simulink model "lab4_test"  (R2016b)
settings: Solver=VariableStepAuto  StartTime=0.0  StopTime=totaltime  RelTol=1e-3
undefined symbols (not defined in the file or in its folder): h, st
libraries: xbsIndex_r4 x1157
(part 2 of 3)

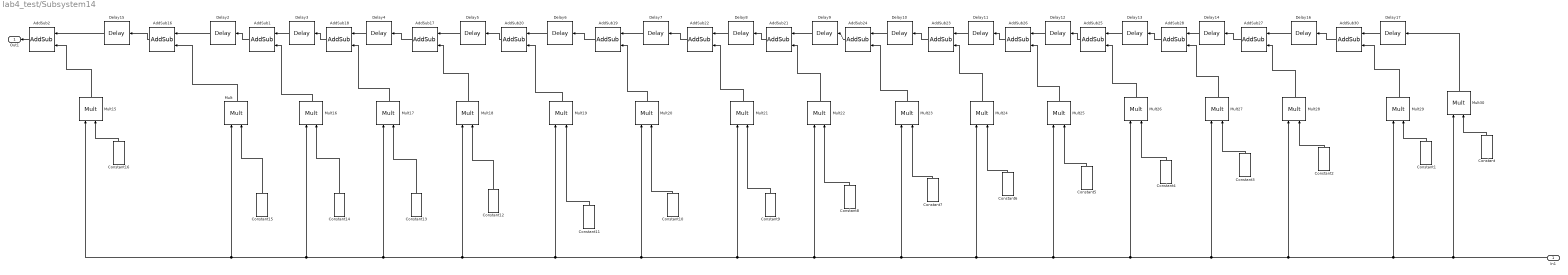
== system lab4_test/Subsystem14 ==
  In1 : Inport
  AddSub{1..2,16..28,30} (16 alike) : xbsIndex_r4/AddSub  mode=Addition  use_carryin=off  use_carryout=off  en=off  latency=0  precision=User Defined  arith_type="Signed  (2's comp)"  n_bits=W  bin_pt=B  quantization=Truncate  overflow=Wrap  use_behavioral_HDL=off  hw_selection=Fabric  pipelined=off  dbl_ovrd=off  block_type=addsub
  Constant : xbsIndex_r4/Constant  const=h(1,4)  gui_display_data_type=Fixed-point  arith_type=Signed (2's comp)  n_bits=W  bin_pt=B  preci_type=Single  exp_width=8  frac_width=24  explicit_period=off  period=1  equ=P=C  opselect=C  inp2=PCIN>>17  opr=+  inp1=P  carry=CIN  dbl_ovrd=off  block_type=constant
  Constant1 : xbsIndex_r4/Constant  const=h(2,4)  gui_display_data_type=Fixed-point  arith_type=Signed (2's comp)  n_bits=W  bin_pt=B  preci_type=Single  exp_width=8  frac_width=24  explicit_period=off  period=1  equ=P=C  opselect=C  inp2=PCIN>>17  opr=+  inp1=P  carry=CIN  dbl_ovrd=off  block_type=constant
  Constant10 : xbsIndex_r4/Constant  const=h(11,4)  gui_display_data_type=Fixed-point  arith_type=Signed (2's comp)  n_bits=W  bin_pt=B  preci_type=Single  exp_width=8  frac_width=24  explicit_period=off  period=1  equ=P=C  opselect=C  inp2=PCIN>>17  opr=+  inp1=P  carry=CIN  dbl_ovrd=off  block_type=constant
  Constant11 : xbsIndex_r4/Constant  const=h(12,4)  gui_display_data_type=Fixed-point  arith_type=Signed (2's comp)  n_bits=W  bin_pt=B  preci_type=Single  exp_width=8  frac_width=24  explicit_period=off  period=1  equ=P=C  opselect=C  inp2=PCIN>>17  opr=+  inp1=P  carry=CIN  dbl_ovrd=off  block_type=constant
  Constant12 : xbsIndex_r4/Constant  const=h(13,4)  gui_display_data_type=Fixed-point  arith_type=Signed (2's comp)  n_bits=W  bin_pt=B  preci_type=Single  exp_width=8  frac_width=24  explicit_period=off  period=1  equ=P=C  opselect=C  inp2=PCIN>>17  opr=+  inp1=P  carry=CIN  dbl_ovrd=off  block_type=constant
  Constant13 : xbsIndex_r4/Constant  const=h(14,4)  gui_display_data_type=Fixed-point  arith_type=Signed (2's comp)  n_bits=W  bin_pt=B  preci_type=Single  exp_width=8  frac_width=24  explicit_period=off  period=1  equ=P=C  opselect=C  inp2=PCIN>>17  opr=+  inp1=P  carry=CIN  dbl_ovrd=off  block_type=constant
  Constant14 : xbsIndex_r4/Constant  const=h(15,4)  gui_display_data_type=Fixed-point  arith_type=Signed (2's comp)  n_bits=W  bin_pt=B  preci_type=Single  exp_width=8  frac_width=24  explicit_period=off  period=1  equ=P=C  opselect=C  inp2=PCIN>>17  opr=+  inp1=P  carry=CIN  dbl_ovrd=off  block_type=constant
  Constant15 : xbsIndex_r4/Constant  const=h(16,4)  gui_display_data_type=Fixed-point  arith_type=Signed (2's comp)  n_bits=W  bin_pt=B  preci_type=Single  exp_width=8  frac_width=24  explicit_period=off  period=1  equ=P=C  opselect=C  inp2=PCIN>>17  opr=+  inp1=P  carry=CIN  dbl_ovrd=off  block_type=constant
  Constant16 : xbsIndex_r4/Constant  const=h(17,4)  gui_display_data_type=Fixed-point  arith_type=Signed (2's comp)  n_bits=W  bin_pt=B  preci_type=Single  exp_width=8  frac_width=24  explicit_period=off  period=1  equ=P=C  opselect=C  inp2=PCIN>>17  opr=+  inp1=P  carry=CIN  dbl_ovrd=off  block_type=constant
  Constant2 : xbsIndex_r4/Constant  const=h(3,4)  gui_display_data_type=Fixed-point  arith_type=Signed (2's comp)  n_bits=W  bin_pt=B  preci_type=Single  exp_width=8  frac_width=24  explicit_period=off  period=1  equ=P=C  opselect=C  inp2=PCIN>>17  opr=+  inp1=P  carry=CIN  dbl_ovrd=off  block_type=constant
  Constant3 : xbsIndex_r4/Constant  const=h(4,4)  gui_display_data_type=Fixed-point  arith_type=Signed (2's comp)  n_bits=W  bin_pt=B  preci_type=Single  exp_width=8  frac_width=24  explicit_period=off  period=1  equ=P=C  opselect=C  inp2=PCIN>>17  opr=+  inp1=P  carry=CIN  dbl_ovrd=off  block_type=constant
  Constant4 : xbsIndex_r4/Constant  const=h(5,4)  gui_display_data_type=Fixed-point  arith_type=Signed (2's comp)  n_bits=W  bin_pt=B  preci_type=Single  exp_width=8  frac_width=24  explicit_period=off  period=1  equ=P=C  opselect=C  inp2=PCIN>>17  opr=+  inp1=P  carry=CIN  dbl_ovrd=off  block_type=constant
  Constant5 : xbsIndex_r4/Constant  const=h(6,4)  gui_display_data_type=Fixed-point  arith_type=Signed (2's comp)  n_bits=W  bin_pt=B  preci_type=Single  exp_width=8  frac_width=24  explicit_period=off  period=1  equ=P=C  opselect=C  inp2=PCIN>>17  opr=+  inp1=P  carry=CIN  dbl_ovrd=off  block_type=constant
  Constant6 : xbsIndex_r4/Constant  const=h(7,4)  gui_display_data_type=Fixed-point  arith_type=Signed (2's comp)  n_bits=W  bin_pt=B  preci_type=Single  exp_width=8  frac_width=24  explicit_period=off  period=1  equ=P=C  opselect=C  inp2=PCIN>>17  opr=+  inp1=P  carry=CIN  dbl_ovrd=off  block_type=constant
  Constant7 : xbsIndex_r4/Constant  const=h(8,4)  gui_display_data_type=Fixed-point  arith_type=Signed (2's comp)  n_bits=W  bin_pt=B  preci_type=Single  exp_width=8  frac_width=24  explicit_period=off  period=1  equ=P=C  opselect=C  inp2=PCIN>>17  opr=+  inp1=P  carry=CIN  dbl_ovrd=off  block_type=constant
  Constant8 : xbsIndex_r4/Constant  const=h(9,4)  gui_display_data_type=Fixed-point  arith_type=Signed (2's comp)  n_bits=W  bin_pt=B  preci_type=Single  exp_width=8  frac_width=24  explicit_period=off  period=1  equ=P=C  opselect=C  inp2=PCIN>>17  opr=+  inp1=P  carry=CIN  dbl_ovrd=off  block_type=constant
  Constant9 : xbsIndex_r4/Constant  const=h(10,4)  gui_display_data_type=Fixed-point  arith_type=Signed (2's comp)  n_bits=W  bin_pt=B  preci_type=Single  exp_width=8  frac_width=24  explicit_period=off  period=1  equ=P=C  opselect=C  inp2=PCIN>>17  opr=+  inp1=P  carry=CIN  dbl_ovrd=off  block_type=constant
  Delay{2..17} (16 alike) : xbsIndex_r4/Delay  rst=off  infoeditControl=Selection of Reset will increase slice count due to use of real FFs and instead of SRLs  en=off  latency=1  reg_retiming=off  dbl_ovrd=off  block_type=delay
  Mult{,15..30} (17 alike) : xbsIndex_r4/Mult  precision=User Defined  arith_type="Signed  (2's comp)"  n_bits=W  bin_pt=B  quantization="Round  (unbiased: +/- Inf)"  overflow=Flag as error  en=off  latency=0  use_behavioral_HDL=off  opt=Speed  use_embedded=on  optimum_pipeline=off  pipeline=on  dbl_ovrd=off  use_rpm=on  placement_style=Triangular  block_type=mult
  Out1 : Outport
  wires:
  AddSub2/1 -> Out1/1
  Constant14/1 -> Mult16/2
  Mult/1 -> AddSub16/2
  Mult16/1 -> AddSub1/2
  AddSub16/1 -> Delay15/1
  Constant15/1 -> Mult/2
  AddSub1/1 -> Delay2/1
  Constant13/1 -> Mult17/2
  Mult17/1 -> AddSub18/2
  Constant12/1 -> Mult18/2
  AddSub17/1 -> Delay4/1
  AddSub18/1 -> Delay3/1
  Constant11/1 -> Mult19/2
  Mult19/1 -> AddSub20/2
  Constant10/1 -> Mult20/2
  Mult20/1 -> AddSub19/2
  AddSub19/1 -> Delay6/1
  AddSub20/1 -> Delay5/1
  Constant9/1 -> Mult21/2
  Mult21/1 -> AddSub22/2
  Constant8/1 -> Mult22/2
  AddSub21/1 -> Delay8/1
  AddSub22/1 -> Delay7/1
  Constant7/1 -> Mult23/2
  Mult23/1 -> AddSub24/2
  Constant6/1 -> Mult24/2
  AddSub23/1 -> Delay10/1
  Constant5/1 -> Mult25/2
  Mult25/1 -> AddSub26/2
  Constant4/1 -> Mult26/2
  Mult26/1 -> AddSub25/2
  AddSub25/1 -> Delay12/1
  AddSub26/1 -> Delay11/1
  Constant3/1 -> Mult27/2
  Mult27/1 -> AddSub28/2
  Constant2/1 -> Mult28/2
  AddSub27/1 -> Delay14/1
  AddSub28/1 -> Delay13/1
  Constant1/1 -> Mult29/2
  Mult29/1 -> AddSub30/2
  Constant/1 -> Mult30/2
  Mult30/1 -> Delay17/1
  AddSub30/1 -> Delay16/1
  AddSub24/1 -> Delay9/1
  Delay2/1 -> AddSub16/1
  Delay3/1 -> AddSub1/1
  Delay4/1 -> AddSub18/1
  Delay6/1 -> AddSub20/1
  Delay7/1 -> AddSub19/1
  Delay8/1 -> AddSub22/1
  Delay10/1 -> AddSub24/1
  Delay12/1 -> AddSub26/1
  Delay13/1 -> AddSub25/1
  Delay14/1 -> AddSub28/1
  Delay17/1 -> AddSub30/1
  Constant16/1 -> Mult15/2
  Mult15/1 -> AddSub2/2
  Delay15/1 -> AddSub2/1
  Delay5/1 -> AddSub17/1
  Mult18/1 -> AddSub17/2
  Delay9/1 -> AddSub21/1
  Mult22/1 -> AddSub21/2
  Delay11/1 -> AddSub23/1
  Mult24/1 -> AddSub23/2
  Delay16/1 -> AddSub27/1
  Mult28/1 -> AddSub27/2
  In1/1 -> Mult30/1, Mult29/1, Mult28/1, Mult27/1, Mult26/1, Mult25/1, Mult24/1, Mult22/1, Mult21/1, Mult19/1, Mult17/1, Mult15/1, Mult/1, Mult16/1, Mult18/1, Mult20/1, Mult23/1

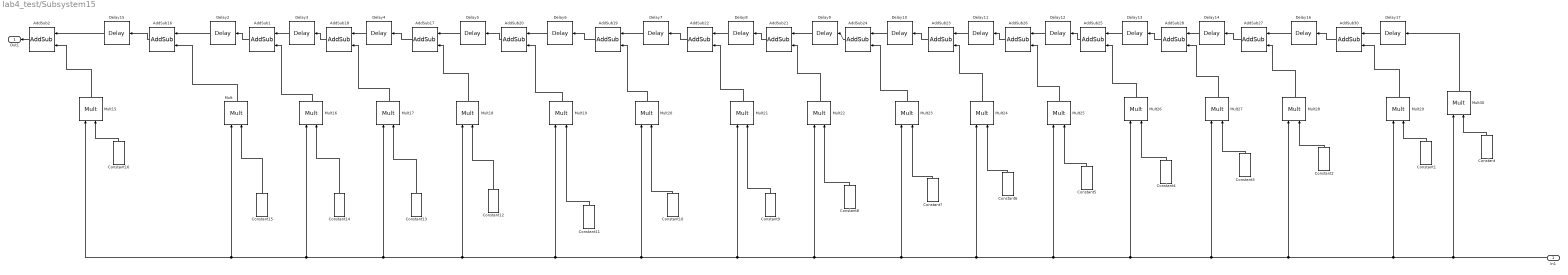
== system lab4_test/Subsystem15 ==
  In1 : Inport
  AddSub{1..2,16..28,30} (16 alike) : xbsIndex_r4/AddSub  mode=Addition  use_carryin=off  use_carryout=off  en=off  latency=0  precision=User Defined  arith_type="Signed  (2's comp)"  n_bits=W  bin_pt=B  quantization=Truncate  overflow=Wrap  use_behavioral_HDL=off  hw_selection=Fabric  pipelined=off  dbl_ovrd=off  block_type=addsub
  Constant : xbsIndex_r4/Constant  const=h(1,3)  gui_display_data_type=Fixed-point  arith_type=Signed (2's comp)  n_bits=W  bin_pt=B  preci_type=Single  exp_width=8  frac_width=24  explicit_period=off  period=1  equ=P=C  opselect=C  inp2=PCIN>>17  opr=+  inp1=P  carry=CIN  dbl_ovrd=off  block_type=constant
  Constant1 : xbsIndex_r4/Constant  const=h(2,3)  gui_display_data_type=Fixed-point  arith_type=Signed (2's comp)  n_bits=W  bin_pt=B  preci_type=Single  exp_width=8  frac_width=24  explicit_period=off  period=1  equ=P=C  opselect=C  inp2=PCIN>>17  opr=+  inp1=P  carry=CIN  dbl_ovrd=off  block_type=constant
  Constant10 : xbsIndex_r4/Constant  const=h(11,3)  gui_display_data_type=Fixed-point  arith_type=Signed (2's comp)  n_bits=W  bin_pt=B  preci_type=Single  exp_width=8  frac_width=24  explicit_period=off  period=1  equ=P=C  opselect=C  inp2=PCIN>>17  opr=+  inp1=P  carry=CIN  dbl_ovrd=off  block_type=constant
  Constant11 : xbsIndex_r4/Constant  const=h(12,3)  gui_display_data_type=Fixed-point  arith_type=Signed (2's comp)  n_bits=W  bin_pt=B  preci_type=Single  exp_width=8  frac_width=24  explicit_period=off  period=1  equ=P=C  opselect=C  inp2=PCIN>>17  opr=+  inp1=P  carry=CIN  dbl_ovrd=off  block_type=constant
  Constant12 : xbsIndex_r4/Constant  const=h(13,3)  gui_display_data_type=Fixed-point  arith_type=Signed (2's comp)  n_bits=W  bin_pt=B  preci_type=Single  exp_width=8  frac_width=24  explicit_period=off  period=1  equ=P=C  opselect=C  inp2=PCIN>>17  opr=+  inp1=P  carry=CIN  dbl_ovrd=off  block_type=constant
  Constant13 : xbsIndex_r4/Constant  const=h(14,3)  gui_display_data_type=Fixed-point  arith_type=Signed (2's comp)  n_bits=W  bin_pt=B  preci_type=Single  exp_width=8  frac_width=24  explicit_period=off  period=1  equ=P=C  opselect=C  inp2=PCIN>>17  opr=+  inp1=P  carry=CIN  dbl_ovrd=off  block_type=constant
  Constant14 : xbsIndex_r4/Constant  const=h(15,3)  gui_display_data_type=Fixed-point  arith_type=Signed (2's comp)  n_bits=W  bin_pt=B  preci_type=Single  exp_width=8  frac_width=24  explicit_period=off  period=1  equ=P=C  opselect=C  inp2=PCIN>>17  opr=+  inp1=P  carry=CIN  dbl_ovrd=off  block_type=constant
  Constant15 : xbsIndex_r4/Constant  const=h(16,3)  gui_display_data_type=Fixed-point  arith_type=Signed (2's comp)  n_bits=W  bin_pt=B  preci_type=Single  exp_width=8  frac_width=24  explicit_period=off  period=1  equ=P=C  opselect=C  inp2=PCIN>>17  opr=+  inp1=P  carry=CIN  dbl_ovrd=off  block_type=constant
  Constant16 : xbsIndex_r4/Constant  const=h(17,3)  gui_display_data_type=Fixed-point  arith_type=Signed (2's comp)  n_bits=W  bin_pt=B  preci_type=Single  exp_width=8  frac_width=24  explicit_period=off  period=1  equ=P=C  opselect=C  inp2=PCIN>>17  opr=+  inp1=P  carry=CIN  dbl_ovrd=off  block_type=constant
  Constant2 : xbsIndex_r4/Constant  const=h(3,3)  gui_display_data_type=Fixed-point  arith_type=Signed (2's comp)  n_bits=W  bin_pt=B  preci_type=Single  exp_width=8  frac_width=24  explicit_period=off  period=1  equ=P=C  opselect=C  inp2=PCIN>>17  opr=+  inp1=P  carry=CIN  dbl_ovrd=off  block_type=constant
  Constant3 : xbsIndex_r4/Constant  const=h(4,3)  gui_display_data_type=Fixed-point  arith_type=Signed (2's comp)  n_bits=W  bin_pt=B  preci_type=Single  exp_width=8  frac_width=24  explicit_period=off  period=1  equ=P=C  opselect=C  inp2=PCIN>>17  opr=+  inp1=P  carry=CIN  dbl_ovrd=off  block_type=constant
  Constant4 : xbsIndex_r4/Constant  const=h(5,3)  gui_display_data_type=Fixed-point  arith_type=Signed (2's comp)  n_bits=W  bin_pt=B  preci_type=Single  exp_width=8  frac_width=24  explicit_period=off  period=1  equ=P=C  opselect=C  inp2=PCIN>>17  opr=+  inp1=P  carry=CIN  dbl_ovrd=off  block_type=constant
  Constant5 : xbsIndex_r4/Constant  const=h(6,3)  gui_display_data_type=Fixed-point  arith_type=Signed (2's comp)  n_bits=W  bin_pt=B  preci_type=Single  exp_width=8  frac_width=24  explicit_period=off  period=1  equ=P=C  opselect=C  inp2=PCIN>>17  opr=+  inp1=P  carry=CIN  dbl_ovrd=off  block_type=constant
  Constant6 : xbsIndex_r4/Constant  const=h(7,3)  gui_display_data_type=Fixed-point  arith_type=Signed (2's comp)  n_bits=W  bin_pt=B  preci_type=Single  exp_width=8  frac_width=24  explicit_period=off  period=1  equ=P=C  opselect=C  inp2=PCIN>>17  opr=+  inp1=P  carry=CIN  dbl_ovrd=off  block_type=constant
  Constant7 : xbsIndex_r4/Constant  const=h(8,3)  gui_display_data_type=Fixed-point  arith_type=Signed (2's comp)  n_bits=W  bin_pt=B  preci_type=Single  exp_width=8  frac_width=24  explicit_period=off  period=1  equ=P=C  opselect=C  inp2=PCIN>>17  opr=+  inp1=P  carry=CIN  dbl_ovrd=off  block_type=constant
  Constant8 : xbsIndex_r4/Constant  const=h(9,3)  gui_display_data_type=Fixed-point  arith_type=Signed (2's comp)  n_bits=W  bin_pt=B  preci_type=Single  exp_width=8  frac_width=24  explicit_period=off  period=1  equ=P=C  opselect=C  inp2=PCIN>>17  opr=+  inp1=P  carry=CIN  dbl_ovrd=off  block_type=constant
  Constant9 : xbsIndex_r4/Constant  const=h(10,3)  gui_display_data_type=Fixed-point  arith_type=Signed (2's comp)  n_bits=W  bin_pt=B  preci_type=Single  exp_width=8  frac_width=24  explicit_period=off  period=1  equ=P=C  opselect=C  inp2=PCIN>>17  opr=+  inp1=P  carry=CIN  dbl_ovrd=off  block_type=constant
  Delay{2..17} (16 alike) : xbsIndex_r4/Delay  rst=off  infoeditControl=Selection of Reset will increase slice count due to use of real FFs and instead of SRLs  en=off  latency=1  reg_retiming=off  dbl_ovrd=off  block_type=delay
  Mult{,15..30} (17 alike) : xbsIndex_r4/Mult  precision=User Defined  arith_type="Signed  (2's comp)"  n_bits=W  bin_pt=B  quantization="Round  (unbiased: +/- Inf)"  overflow=Flag as error  en=off  latency=0  use_behavioral_HDL=off  opt=Speed  use_embedded=on  optimum_pipeline=off  pipeline=on  dbl_ovrd=off  use_rpm=on  placement_style=Triangular  block_type=mult
  Out1 : Outport
  wires:
  AddSub2/1 -> Out1/1
  Constant14/1 -> Mult16/2
  Mult/1 -> AddSub16/2
  Mult16/1 -> AddSub1/2
  AddSub16/1 -> Delay15/1
  Constant15/1 -> Mult/2
  AddSub1/1 -> Delay2/1
  Constant13/1 -> Mult17/2
  Mult17/1 -> AddSub18/2
  Constant12/1 -> Mult18/2
  AddSub17/1 -> Delay4/1
  AddSub18/1 -> Delay3/1
  Constant11/1 -> Mult19/2
  Mult19/1 -> AddSub20/2
  Constant10/1 -> Mult20/2
  Mult20/1 -> AddSub19/2
  AddSub19/1 -> Delay6/1
  AddSub20/1 -> Delay5/1
  Constant9/1 -> Mult21/2
  Mult21/1 -> AddSub22/2
  Constant8/1 -> Mult22/2
  AddSub21/1 -> Delay8/1
  AddSub22/1 -> Delay7/1
  Constant7/1 -> Mult23/2
  Mult23/1 -> AddSub24/2
  Constant6/1 -> Mult24/2
  AddSub23/1 -> Delay10/1
  Constant5/1 -> Mult25/2
  Mult25/1 -> AddSub26/2
  Constant4/1 -> Mult26/2
  Mult26/1 -> AddSub25/2
  AddSub25/1 -> Delay12/1
  AddSub26/1 -> Delay11/1
  Constant3/1 -> Mult27/2
  Mult27/1 -> AddSub28/2
  Constant2/1 -> Mult28/2
  AddSub27/1 -> Delay14/1
  AddSub28/1 -> Delay13/1
  Constant1/1 -> Mult29/2
  Mult29/1 -> AddSub30/2
  Constant/1 -> Mult30/2
  Mult30/1 -> Delay17/1
  AddSub30/1 -> Delay16/1
  AddSub24/1 -> Delay9/1
  Delay2/1 -> AddSub16/1
  Delay3/1 -> AddSub1/1
  Delay4/1 -> AddSub18/1
  Delay6/1 -> AddSub20/1
  Delay7/1 -> AddSub19/1
  Delay8/1 -> AddSub22/1
  Delay10/1 -> AddSub24/1
  Delay12/1 -> AddSub26/1
  Delay13/1 -> AddSub25/1
  Delay14/1 -> AddSub28/1
  Delay17/1 -> AddSub30/1
  Constant16/1 -> Mult15/2
  Mult15/1 -> AddSub2/2
  Delay15/1 -> AddSub2/1
  Delay5/1 -> AddSub17/1
  Mult18/1 -> AddSub17/2
  Delay9/1 -> AddSub21/1
  Mult22/1 -> AddSub21/2
  Delay11/1 -> AddSub23/1
  Mult24/1 -> AddSub23/2
  Delay16/1 -> AddSub27/1
  Mult28/1 -> AddSub27/2
  In1/1 -> Mult30/1, Mult29/1, Mult28/1, Mult27/1, Mult26/1, Mult25/1, Mult24/1, Mult22/1, Mult21/1, Mult19/1, Mult17/1, Mult15/1, Mult/1, Mult16/1, Mult18/1, Mult20/1, Mult23/1

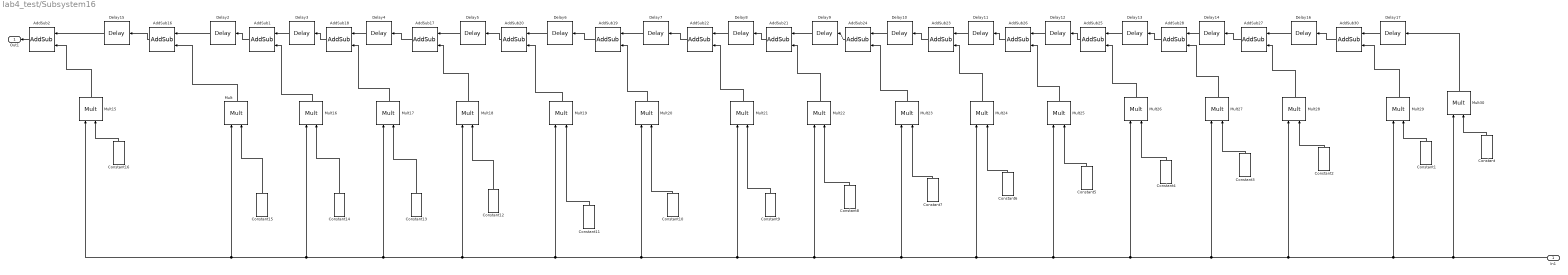
== system lab4_test/Subsystem16 ==
  In1 : Inport
  AddSub{1..2,16..28,30} (16 alike) : xbsIndex_r4/AddSub  mode=Addition  use_carryin=off  use_carryout=off  en=off  latency=0  precision=User Defined  arith_type="Signed  (2's comp)"  n_bits=W  bin_pt=B  quantization=Truncate  overflow=Wrap  use_behavioral_HDL=off  hw_selection=Fabric  pipelined=off  dbl_ovrd=off  block_type=addsub
  Constant : xbsIndex_r4/Constant  const=h(1,2)  gui_display_data_type=Fixed-point  arith_type=Signed (2's comp)  n_bits=W  bin_pt=B  preci_type=Single  exp_width=8  frac_width=24  explicit_period=off  period=1  equ=P=C  opselect=C  inp2=PCIN>>17  opr=+  inp1=P  carry=CIN  dbl_ovrd=off  block_type=constant
  Constant1 : xbsIndex_r4/Constant  const=h(2,2)  gui_display_data_type=Fixed-point  arith_type=Signed (2's comp)  n_bits=W  bin_pt=B  preci_type=Single  exp_width=8  frac_width=24  explicit_period=off  period=1  equ=P=C  opselect=C  inp2=PCIN>>17  opr=+  inp1=P  carry=CIN  dbl_ovrd=off  block_type=constant
  Constant10 : xbsIndex_r4/Constant  const=h(11,2)  gui_display_data_type=Fixed-point  arith_type=Signed (2's comp)  n_bits=W  bin_pt=B  preci_type=Single  exp_width=8  frac_width=24  explicit_period=off  period=1  equ=P=C  opselect=C  inp2=PCIN>>17  opr=+  inp1=P  carry=CIN  dbl_ovrd=off  block_type=constant
  Constant11 : xbsIndex_r4/Constant  const=h(12,2)  gui_display_data_type=Fixed-point  arith_type=Signed (2's comp)  n_bits=W  bin_pt=B  preci_type=Single  exp_width=8  frac_width=24  explicit_period=off  period=1  equ=P=C  opselect=C  inp2=PCIN>>17  opr=+  inp1=P  carry=CIN  dbl_ovrd=off  block_type=constant
  Constant12 : xbsIndex_r4/Constant  const=h(13,2)  gui_display_data_type=Fixed-point  arith_type=Signed (2's comp)  n_bits=W  bin_pt=B  preci_type=Single  exp_width=8  frac_width=24  explicit_period=off  period=1  equ=P=C  opselect=C  inp2=PCIN>>17  opr=+  inp1=P  carry=CIN  dbl_ovrd=off  block_type=constant
  Constant13 : xbsIndex_r4/Constant  const=h(14,2)  gui_display_data_type=Fixed-point  arith_type=Signed (2's comp)  n_bits=W  bin_pt=B  preci_type=Single  exp_width=8  frac_width=24  explicit_period=off  period=1  equ=P=C  opselect=C  inp2=PCIN>>17  opr=+  inp1=P  carry=CIN  dbl_ovrd=off  block_type=constant
  Constant14 : xbsIndex_r4/Constant  const=h(15,2)  gui_display_data_type=Fixed-point  arith_type=Signed (2's comp)  n_bits=W  bin_pt=B  preci_type=Single  exp_width=8  frac_width=24  explicit_period=off  period=1  equ=P=C  opselect=C  inp2=PCIN>>17  opr=+  inp1=P  carry=CIN  dbl_ovrd=off  block_type=constant
  Constant15 : xbsIndex_r4/Constant  const=h(16,2)  gui_display_data_type=Fixed-point  arith_type=Signed (2's comp)  n_bits=W  bin_pt=B  preci_type=Single  exp_width=8  frac_width=24  explicit_period=off  period=1  equ=P=C  opselect=C  inp2=PCIN>>17  opr=+  inp1=P  carry=CIN  dbl_ovrd=off  block_type=constant
  Constant16 : xbsIndex_r4/Constant  const=h(17,2)  gui_display_data_type=Fixed-point  arith_type=Signed (2's comp)  n_bits=W  bin_pt=B  preci_type=Single  exp_width=8  frac_width=24  explicit_period=off  period=1  equ=P=C  opselect=C  inp2=PCIN>>17  opr=+  inp1=P  carry=CIN  dbl_ovrd=off  block_type=constant
  Constant2 : xbsIndex_r4/Constant  const=h(3,2)  gui_display_data_type=Fixed-point  arith_type=Signed (2's comp)  n_bits=W  bin_pt=B  preci_type=Single  exp_width=8  frac_width=24  explicit_period=off  period=1  equ=P=C  opselect=C  inp2=PCIN>>17  opr=+  inp1=P  carry=CIN  dbl_ovrd=off  block_type=constant
  Constant3 : xbsIndex_r4/Constant  const=h(4,2)  gui_display_data_type=Fixed-point  arith_type=Signed (2's comp)  n_bits=W  bin_pt=B  preci_type=Single  exp_width=8  frac_width=24  explicit_period=off  period=1  equ=P=C  opselect=C  inp2=PCIN>>17  opr=+  inp1=P  carry=CIN  dbl_ovrd=off  block_type=constant
  Constant4 : xbsIndex_r4/Constant  const=h(5,2)  gui_display_data_type=Fixed-point  arith_type=Signed (2's comp)  n_bits=W  bin_pt=B  preci_type=Single  exp_width=8  frac_width=24  explicit_period=off  period=1  equ=P=C  opselect=C  inp2=PCIN>>17  opr=+  inp1=P  carry=CIN  dbl_ovrd=off  block_type=constant
  Constant5 : xbsIndex_r4/Constant  const=h(6,2)  gui_display_data_type=Fixed-point  arith_type=Signed (2's comp)  n_bits=W  bin_pt=B  preci_type=Single  exp_width=8  frac_width=24  explicit_period=off  period=1  equ=P=C  opselect=C  inp2=PCIN>>17  opr=+  inp1=P  carry=CIN  dbl_ovrd=off  block_type=constant
  Constant6 : xbsIndex_r4/Constant  const=h(7,2)  gui_display_data_type=Fixed-point  arith_type=Signed (2's comp)  n_bits=W  bin_pt=B  preci_type=Single  exp_width=8  frac_width=24  explicit_period=off  period=1  equ=P=C  opselect=C  inp2=PCIN>>17  opr=+  inp1=P  carry=CIN  dbl_ovrd=off  block_type=constant
  Constant7 : xbsIndex_r4/Constant  const=h(8,2)  gui_display_data_type=Fixed-point  arith_type=Signed (2's comp)  n_bits=W  bin_pt=B  preci_type=Single  exp_width=8  frac_width=24  explicit_period=off  period=1  equ=P=C  opselect=C  inp2=PCIN>>17  opr=+  inp1=P  carry=CIN  dbl_ovrd=off  block_type=constant
  Constant8 : xbsIndex_r4/Constant  const=h(9,2)  gui_display_data_type=Fixed-point  arith_type=Signed (2's comp)  n_bits=W  bin_pt=B  preci_type=Single  exp_width=8  frac_width=24  explicit_period=off  period=1  equ=P=C  opselect=C  inp2=PCIN>>17  opr=+  inp1=P  carry=CIN  dbl_ovrd=off  block_type=constant
  Constant9 : xbsIndex_r4/Constant  const=h(10,2)  gui_display_data_type=Fixed-point  arith_type=Signed (2's comp)  n_bits=W  bin_pt=B  preci_type=Single  exp_width=8  frac_width=24  explicit_period=off  period=1  equ=P=C  opselect=C  inp2=PCIN>>17  opr=+  inp1=P  carry=CIN  dbl_ovrd=off  block_type=constant
  Delay{2..17} (16 alike) : xbsIndex_r4/Delay  rst=off  infoeditControl=Selection of Reset will increase slice count due to use of real FFs and instead of SRLs  en=off  latency=1  reg_retiming=off  dbl_ovrd=off  block_type=delay
  Mult{,15..30} (17 alike) : xbsIndex_r4/Mult  precision=User Defined  arith_type="Signed  (2's comp)"  n_bits=W  bin_pt=B  quantization="Round  (unbiased: +/- Inf)"  overflow=Flag as error  en=off  latency=0  use_behavioral_HDL=off  opt=Speed  use_embedded=on  optimum_pipeline=off  pipeline=on  dbl_ovrd=off  use_rpm=on  placement_style=Triangular  block_type=mult
  Out1 : Outport
  wires:
  AddSub2/1 -> Out1/1
  Constant14/1 -> Mult16/2
  Mult/1 -> AddSub16/2
  Mult16/1 -> AddSub1/2
  AddSub16/1 -> Delay15/1
  Constant15/1 -> Mult/2
  AddSub1/1 -> Delay2/1
  Constant13/1 -> Mult17/2
  Mult17/1 -> AddSub18/2
  Constant12/1 -> Mult18/2
  AddSub17/1 -> Delay4/1
  AddSub18/1 -> Delay3/1
  Constant11/1 -> Mult19/2
  Mult19/1 -> AddSub20/2
  Constant10/1 -> Mult20/2
  Mult20/1 -> AddSub19/2
  AddSub19/1 -> Delay6/1
  AddSub20/1 -> Delay5/1
  Constant9/1 -> Mult21/2
  Mult21/1 -> AddSub22/2
  Constant8/1 -> Mult22/2
  AddSub21/1 -> Delay8/1
  AddSub22/1 -> Delay7/1
  Constant7/1 -> Mult23/2
  Mult23/1 -> AddSub24/2
  Constant6/1 -> Mult24/2
  AddSub23/1 -> Delay10/1
  Constant5/1 -> Mult25/2
  Mult25/1 -> AddSub26/2
  Constant4/1 -> Mult26/2
  Mult26/1 -> AddSub25/2
  AddSub25/1 -> Delay12/1
  AddSub26/1 -> Delay11/1
  Constant3/1 -> Mult27/2
  Mult27/1 -> AddSub28/2
  Constant2/1 -> Mult28/2
  AddSub27/1 -> Delay14/1
  AddSub28/1 -> Delay13/1
  Constant1/1 -> Mult29/2
  Mult29/1 -> AddSub30/2
  Constant/1 -> Mult30/2
  Mult30/1 -> Delay17/1
  AddSub30/1 -> Delay16/1
  AddSub24/1 -> Delay9/1
  Delay2/1 -> AddSub16/1
  Delay3/1 -> AddSub1/1
  Delay4/1 -> AddSub18/1
  Delay6/1 -> AddSub20/1
  Delay7/1 -> AddSub19/1
  Delay8/1 -> AddSub22/1
  Delay10/1 -> AddSub24/1
  Delay12/1 -> AddSub26/1
  Delay13/1 -> AddSub25/1
  Delay14/1 -> AddSub28/1
  Delay17/1 -> AddSub30/1
  Constant16/1 -> Mult15/2
  Mult15/1 -> AddSub2/2
  Delay15/1 -> AddSub2/1
  Delay5/1 -> AddSub17/1
  Mult18/1 -> AddSub17/2
  Delay9/1 -> AddSub21/1
  Mult22/1 -> AddSub21/2
  Delay11/1 -> AddSub23/1
  Mult24/1 -> AddSub23/2
  Delay16/1 -> AddSub27/1
  Mult28/1 -> AddSub27/2
  In1/1 -> Mult30/1, Mult29/1, Mult28/1, Mult27/1, Mult26/1, Mult25/1, Mult24/1, Mult22/1, Mult21/1, Mult19/1, Mult17/1, Mult15/1, Mult/1, Mult16/1, Mult18/1, Mult20/1, Mult23/1

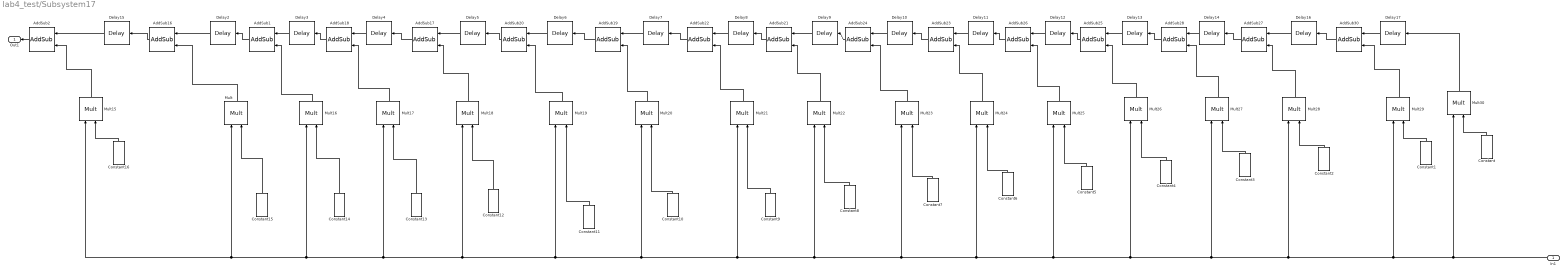
== system lab4_test/Subsystem17 ==
  In1 : Inport
  AddSub{1..2,16..28,30} (16 alike) : xbsIndex_r4/AddSub  mode=Addition  use_carryin=off  use_carryout=off  en=off  latency=0  precision=User Defined  arith_type="Signed  (2's comp)"  n_bits=W  bin_pt=B  quantization=Truncate  overflow=Wrap  use_behavioral_HDL=off  hw_selection=Fabric  pipelined=off  dbl_ovrd=off  block_type=addsub
  Constant : xbsIndex_r4/Constant  const=h(1,1)  gui_display_data_type=Fixed-point  arith_type=Signed (2's comp)  n_bits=W  bin_pt=B  preci_type=Single  exp_width=8  frac_width=24  explicit_period=off  period=1  equ=P=C  opselect=C  inp2=PCIN>>17  opr=+  inp1=P  carry=CIN  dbl_ovrd=off  block_type=constant
  Constant1 : xbsIndex_r4/Constant  const=h(2,1)  gui_display_data_type=Fixed-point  arith_type=Signed (2's comp)  n_bits=W  bin_pt=B  preci_type=Single  exp_width=8  frac_width=24  explicit_period=off  period=1  equ=P=C  opselect=C  inp2=PCIN>>17  opr=+  inp1=P  carry=CIN  dbl_ovrd=off  block_type=constant
  Constant10 : xbsIndex_r4/Constant  const=h(11,1)  gui_display_data_type=Fixed-point  arith_type=Signed (2's comp)  n_bits=W  bin_pt=B  preci_type=Single  exp_width=8  frac_width=24  explicit_period=off  period=1  equ=P=C  opselect=C  inp2=PCIN>>17  opr=+  inp1=P  carry=CIN  dbl_ovrd=off  block_type=constant
  Constant11 : xbsIndex_r4/Constant  const=h(12,1)  gui_display_data_type=Fixed-point  arith_type=Signed (2's comp)  n_bits=W  bin_pt=B  preci_type=Single  exp_width=8  frac_width=24  explicit_period=off  period=1  equ=P=C  opselect=C  inp2=PCIN>>17  opr=+  inp1=P  carry=CIN  dbl_ovrd=off  block_type=constant
  Constant12 : xbsIndex_r4/Constant  const=h(13,1)  gui_display_data_type=Fixed-point  arith_type=Signed (2's comp)  n_bits=W  bin_pt=B  preci_type=Single  exp_width=8  frac_width=24  explicit_period=off  period=1  equ=P=C  opselect=C  inp2=PCIN>>17  opr=+  inp1=P  carry=CIN  dbl_ovrd=off  block_type=constant
  Constant13 : xbsIndex_r4/Constant  const=h(14,1)  gui_display_data_type=Fixed-point  arith_type=Signed (2's comp)  n_bits=W  bin_pt=B  preci_type=Single  exp_width=8  frac_width=24  explicit_period=off  period=1  equ=P=C  opselect=C  inp2=PCIN>>17  opr=+  inp1=P  carry=CIN  dbl_ovrd=off  block_type=constant
  Constant14 : xbsIndex_r4/Constant  const=h(15,1)  gui_display_data_type=Fixed-point  arith_type=Signed (2's comp)  n_bits=W  bin_pt=B  preci_type=Single  exp_width=8  frac_width=24  explicit_period=off  period=1  equ=P=C  opselect=C  inp2=PCIN>>17  opr=+  inp1=P  carry=CIN  dbl_ovrd=off  block_type=constant
  Constant15 : xbsIndex_r4/Constant  const=h(16,1)  gui_display_data_type=Fixed-point  arith_type=Signed (2's comp)  n_bits=W  bin_pt=B  preci_type=Single  exp_width=8  frac_width=24  explicit_period=off  period=1  equ=P=C  opselect=C  inp2=PCIN>>17  opr=+  inp1=P  carry=CIN  dbl_ovrd=off  block_type=constant
  Constant16 : xbsIndex_r4/Constant  const=h(17,1)  gui_display_data_type=Fixed-point  arith_type=Signed (2's comp)  n_bits=W  bin_pt=B  preci_type=Single  exp_width=8  frac_width=24  explicit_period=off  period=1  equ=P=C  opselect=C  inp2=PCIN>>17  opr=+  inp1=P  carry=CIN  dbl_ovrd=off  block_type=constant
  Constant2 : xbsIndex_r4/Constant  const=h(3,1)  gui_display_data_type=Fixed-point  arith_type=Signed (2's comp)  n_bits=W  bin_pt=B  preci_type=Single  exp_width=8  frac_width=24  explicit_period=off  period=1  equ=P=C  opselect=C  inp2=PCIN>>17  opr=+  inp1=P  carry=CIN  dbl_ovrd=off  block_type=constant
  Constant3 : xbsIndex_r4/Constant  const=h(4,1)  gui_display_data_type=Fixed-point  arith_type=Signed (2's comp)  n_bits=W  bin_pt=B  preci_type=Single  exp_width=8  frac_width=24  explicit_period=off  period=1  equ=P=C  opselect=C  inp2=PCIN>>17  opr=+  inp1=P  carry=CIN  dbl_ovrd=off  block_type=constant
  Constant4 : xbsIndex_r4/Constant  const=h(5,1)  gui_display_data_type=Fixed-point  arith_type=Signed (2's comp)  n_bits=W  bin_pt=B  preci_type=Single  exp_width=8  frac_width=24  explicit_period=off  period=1  equ=P=C  opselect=C  inp2=PCIN>>17  opr=+  inp1=P  carry=CIN  dbl_ovrd=off  block_type=constant
  Constant5 : xbsIndex_r4/Constant  const=h(6,1)  gui_display_data_type=Fixed-point  arith_type=Signed (2's comp)  n_bits=W  bin_pt=B  preci_type=Single  exp_width=8  frac_width=24  explicit_period=off  period=1  equ=P=C  opselect=C  inp2=PCIN>>17  opr=+  inp1=P  carry=CIN  dbl_ovrd=off  block_type=constant
  Constant6 : xbsIndex_r4/Constant  const=h(7,1)  gui_display_data_type=Fixed-point  arith_type=Signed (2's comp)  n_bits=W  bin_pt=B  preci_type=Single  exp_width=8  frac_width=24  explicit_period=off  period=1  equ=P=C  opselect=C  inp2=PCIN>>17  opr=+  inp1=P  carry=CIN  dbl_ovrd=off  block_type=constant
  Constant7 : xbsIndex_r4/Constant  const=h(8,1)  gui_display_data_type=Fixed-point  arith_type=Signed (2's comp)  n_bits=W  bin_pt=B  preci_type=Single  exp_width=8  frac_width=24  explicit_period=off  period=1  equ=P=C  opselect=C  inp2=PCIN>>17  opr=+  inp1=P  carry=CIN  dbl_ovrd=off  block_type=constant
  Constant8 : xbsIndex_r4/Constant  const=h(9,1)  gui_display_data_type=Fixed-point  arith_type=Signed (2's comp)  n_bits=W  bin_pt=B  preci_type=Single  exp_width=8  frac_width=24  explicit_period=off  period=1  equ=P=C  opselect=C  inp2=PCIN>>17  opr=+  inp1=P  carry=CIN  dbl_ovrd=off  block_type=constant
  Constant9 : xbsIndex_r4/Constant  const=h(10,1)  gui_display_data_type=Fixed-point  arith_type=Signed (2's comp)  n_bits=W  bin_pt=B  preci_type=Single  exp_width=8  frac_width=24  explicit_period=off  period=1  equ=P=C  opselect=C  inp2=PCIN>>17  opr=+  inp1=P  carry=CIN  dbl_ovrd=off  block_type=constant
  Delay{2..17} (16 alike) : xbsIndex_r4/Delay  rst=off  infoeditControl=Selection of Reset will increase slice count due to use of real FFs and instead of SRLs  en=off  latency=1  reg_retiming=off  dbl_ovrd=off  block_type=delay
  Mult{,15..30} (17 alike) : xbsIndex_r4/Mult  precision=User Defined  arith_type="Signed  (2's comp)"  n_bits=W  bin_pt=B  quantization="Round  (unbiased: +/- Inf)"  overflow=Flag as error  en=off  latency=0  use_behavioral_HDL=off  opt=Speed  use_embedded=on  optimum_pipeline=off  pipeline=on  dbl_ovrd=off  use_rpm=on  placement_style=Triangular  block_type=mult
  Out1 : Outport
  wires:
  AddSub2/1 -> Out1/1
  Constant14/1 -> Mult16/2
  Mult/1 -> AddSub16/2
  Mult16/1 -> AddSub1/2
  AddSub16/1 -> Delay15/1
  Constant15/1 -> Mult/2
  AddSub1/1 -> Delay2/1
  Constant13/1 -> Mult17/2
  Mult17/1 -> AddSub18/2
  Constant12/1 -> Mult18/2
  AddSub17/1 -> Delay4/1
  AddSub18/1 -> Delay3/1
  Constant11/1 -> Mult19/2
  Mult19/1 -> AddSub20/2
  Constant10/1 -> Mult20/2
  Mult20/1 -> AddSub19/2
  AddSub19/1 -> Delay6/1
  AddSub20/1 -> Delay5/1
  Constant9/1 -> Mult21/2
  Mult21/1 -> AddSub22/2
  Constant8/1 -> Mult22/2
  AddSub21/1 -> Delay8/1
  AddSub22/1 -> Delay7/1
  Constant7/1 -> Mult23/2
  Mult23/1 -> AddSub24/2
  Constant6/1 -> Mult24/2
  AddSub23/1 -> Delay10/1
  Constant5/1 -> Mult25/2
  Mult25/1 -> AddSub26/2
  Constant4/1 -> Mult26/2
  Mult26/1 -> AddSub25/2
  AddSub25/1 -> Delay12/1
  AddSub26/1 -> Delay11/1
  Constant3/1 -> Mult27/2
  Mult27/1 -> AddSub28/2
  Constant2/1 -> Mult28/2
  AddSub27/1 -> Delay14/1
  AddSub28/1 -> Delay13/1
  Constant1/1 -> Mult29/2
  Mult29/1 -> AddSub30/2
  Constant/1 -> Mult30/2
  Mult30/1 -> Delay17/1
  AddSub30/1 -> Delay16/1
  AddSub24/1 -> Delay9/1
  Delay2/1 -> AddSub16/1
  Delay3/1 -> AddSub1/1
  Delay4/1 -> AddSub18/1
  Delay6/1 -> AddSub20/1
  Delay7/1 -> AddSub19/1
  Delay8/1 -> AddSub22/1
  Delay10/1 -> AddSub24/1
  Delay12/1 -> AddSub26/1
  Delay13/1 -> AddSub25/1
  Delay14/1 -> AddSub28/1
  Delay17/1 -> AddSub30/1
  Constant16/1 -> Mult15/2
  Mult15/1 -> AddSub2/2
  Delay15/1 -> AddSub2/1
  Delay5/1 -> AddSub17/1
  Mult18/1 -> AddSub17/2
  Delay9/1 -> AddSub21/1
  Mult22/1 -> AddSub21/2
  Delay11/1 -> AddSub23/1
  Mult24/1 -> AddSub23/2
  Delay16/1 -> AddSub27/1
  Mult28/1 -> AddSub27/2
  In1/1 -> Mult30/1, Mult29/1, Mult28/1, Mult27/1, Mult26/1, Mult25/1, Mult24/1, Mult22/1, Mult21/1, Mult19/1, Mult17/1, Mult15/1, Mult/1, Mult16/1, Mult18/1, Mult20/1, Mult23/1

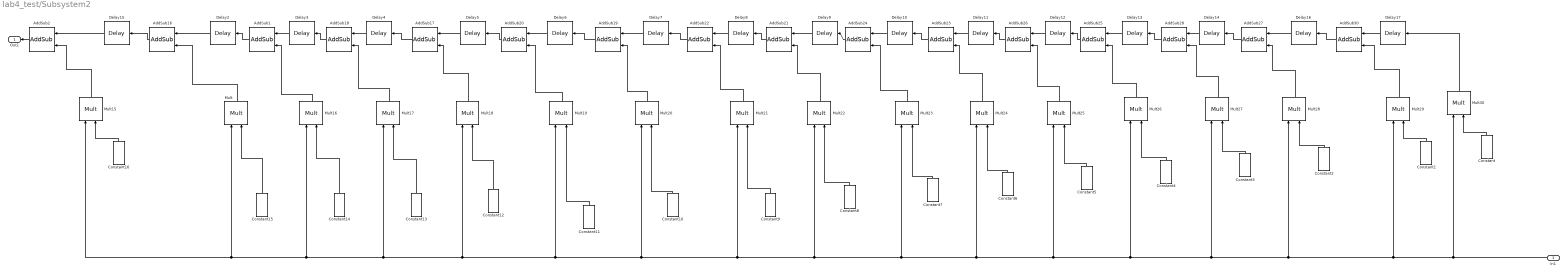
== system lab4_test/Subsystem2 ==
  In1 : Inport
  AddSub{1..2,16..28,30} (16 alike) : xbsIndex_r4/AddSub  mode=Addition  use_carryin=off  use_carryout=off  en=off  latency=0  precision=User Defined  arith_type="Signed  (2's comp)"  n_bits=W  bin_pt=B  quantization=Truncate  overflow=Wrap  use_behavioral_HDL=off  hw_selection=Fabric  pipelined=off  dbl_ovrd=off  block_type=addsub
  Constant : xbsIndex_r4/Constant  const=h(1,16)  gui_display_data_type=Fixed-point  arith_type=Signed (2's comp)  n_bits=W  bin_pt=B  preci_type=Single  exp_width=8  frac_width=24  explicit_period=off  period=1  equ=P=C  opselect=C  inp2=PCIN>>17  opr=+  inp1=P  carry=CIN  dbl_ovrd=off  block_type=constant
  Constant1 : xbsIndex_r4/Constant  const=h(2,16)  gui_display_data_type=Fixed-point  arith_type=Signed (2's comp)  n_bits=W  bin_pt=B  preci_type=Single  exp_width=8  frac_width=24  explicit_period=off  period=1  equ=P=C  opselect=C  inp2=PCIN>>17  opr=+  inp1=P  carry=CIN  dbl_ovrd=off  block_type=constant
  Constant10 : xbsIndex_r4/Constant  const=h(11,16)  gui_display_data_type=Fixed-point  arith_type=Signed (2's comp)  n_bits=W  bin_pt=B  preci_type=Single  exp_width=8  frac_width=24  explicit_period=off  period=1  equ=P=C  opselect=C  inp2=PCIN>>17  opr=+  inp1=P  carry=CIN  dbl_ovrd=off  block_type=constant
  Constant11 : xbsIndex_r4/Constant  const=h(12,16)  gui_display_data_type=Fixed-point  arith_type=Signed (2's comp)  n_bits=W  bin_pt=B  preci_type=Single  exp_width=8  frac_width=24  explicit_period=off  period=1  equ=P=C  opselect=C  inp2=PCIN>>17  opr=+  inp1=P  carry=CIN  dbl_ovrd=off  block_type=constant
  Constant12 : xbsIndex_r4/Constant  const=h(13,16)  gui_display_data_type=Fixed-point  arith_type=Signed (2's comp)  n_bits=W  bin_pt=B  preci_type=Single  exp_width=8  frac_width=24  explicit_period=off  period=1  equ=P=C  opselect=C  inp2=PCIN>>17  opr=+  inp1=P  carry=CIN  dbl_ovrd=off  block_type=constant
  Constant13 : xbsIndex_r4/Constant  const=h(14,16)  gui_display_data_type=Fixed-point  arith_type=Signed (2's comp)  n_bits=W  bin_pt=B  preci_type=Single  exp_width=8  frac_width=24  explicit_period=off  period=1  equ=P=C  opselect=C  inp2=PCIN>>17  opr=+  inp1=P  carry=CIN  dbl_ovrd=off  block_type=constant
  Constant14 : xbsIndex_r4/Constant  const=h(15,16)  gui_display_data_type=Fixed-point  arith_type=Signed (2's comp)  n_bits=W  bin_pt=B  preci_type=Single  exp_width=8  frac_width=24  explicit_period=off  period=1  equ=P=C  opselect=C  inp2=PCIN>>17  opr=+  inp1=P  carry=CIN  dbl_ovrd=off  block_type=constant
  Constant15 : xbsIndex_r4/Constant  const=h(16,16)  gui_display_data_type=Fixed-point  arith_type=Signed (2's comp)  n_bits=W  bin_pt=B  preci_type=Single  exp_width=8  frac_width=24  explicit_period=off  period=1  equ=P=C  opselect=C  inp2=PCIN>>17  opr=+  inp1=P  carry=CIN  dbl_ovrd=off  block_type=constant
  Constant16 : xbsIndex_r4/Constant  const=h(17,16)  gui_display_data_type=Fixed-point  arith_type=Signed (2's comp)  n_bits=W  bin_pt=B  preci_type=Single  exp_width=8  frac_width=24  explicit_period=off  period=1  equ=P=C  opselect=C  inp2=PCIN>>17  opr=+  inp1=P  carry=CIN  dbl_ovrd=off  block_type=constant
  Constant2 : xbsIndex_r4/Constant  const=h(3,16)  gui_display_data_type=Fixed-point  arith_type=Signed (2's comp)  n_bits=W  bin_pt=B  preci_type=Single  exp_width=8  frac_width=24  explicit_period=off  period=1  equ=P=C  opselect=C  inp2=PCIN>>17  opr=+  inp1=P  carry=CIN  dbl_ovrd=off  block_type=constant
  Constant3 : xbsIndex_r4/Constant  const=h(4,16)  gui_display_data_type=Fixed-point  arith_type=Signed (2's comp)  n_bits=W  bin_pt=B  preci_type=Single  exp_width=8  frac_width=24  explicit_period=off  period=1  equ=P=C  opselect=C  inp2=PCIN>>17  opr=+  inp1=P  carry=CIN  dbl_ovrd=off  block_type=constant
  Constant4 : xbsIndex_r4/Constant  const=h(5,16)  gui_display_data_type=Fixed-point  arith_type=Signed (2's comp)  n_bits=W  bin_pt=B  preci_type=Single  exp_width=8  frac_width=24  explicit_period=off  period=1  equ=P=C  opselect=C  inp2=PCIN>>17  opr=+  inp1=P  carry=CIN  dbl_ovrd=off  block_type=constant
  Constant5 : xbsIndex_r4/Constant  const=h(6,16)  gui_display_data_type=Fixed-point  arith_type=Signed (2's comp)  n_bits=W  bin_pt=B  preci_type=Single  exp_width=8  frac_width=24  explicit_period=off  period=1  equ=P=C  opselect=C  inp2=PCIN>>17  opr=+  inp1=P  carry=CIN  dbl_ovrd=off  block_type=constant
  Constant6 : xbsIndex_r4/Constant  const=h(7,16)  gui_display_data_type=Fixed-point  arith_type=Signed (2's comp)  n_bits=W  bin_pt=B  preci_type=Single  exp_width=8  frac_width=24  explicit_period=off  period=1  equ=P=C  opselect=C  inp2=PCIN>>17  opr=+  inp1=P  carry=CIN  dbl_ovrd=off  block_type=constant
  Constant7 : xbsIndex_r4/Constant  const=h(8,16)  gui_display_data_type=Fixed-point  arith_type=Signed (2's comp)  n_bits=W  bin_pt=B  preci_type=Single  exp_width=8  frac_width=24  explicit_period=off  period=1  equ=P=C  opselect=C  inp2=PCIN>>17  opr=+  inp1=P  carry=CIN  dbl_ovrd=off  block_type=constant
  Constant8 : xbsIndex_r4/Constant  const=h(9,16)  gui_display_data_type=Fixed-point  arith_type=Signed (2's comp)  n_bits=W  bin_pt=B  preci_type=Single  exp_width=8  frac_width=24  explicit_period=off  period=1  equ=P=C  opselect=C  inp2=PCIN>>17  opr=+  inp1=P  carry=CIN  dbl_ovrd=off  block_type=constant
  Constant9 : xbsIndex_r4/Constant  const=h(10,16)  gui_display_data_type=Fixed-point  arith_type=Signed (2's comp)  n_bits=W  bin_pt=B  preci_type=Single  exp_width=8  frac_width=24  explicit_period=off  period=1  equ=P=C  opselect=C  inp2=PCIN>>17  opr=+  inp1=P  carry=CIN  dbl_ovrd=off  block_type=constant
  Delay{2..17} (16 alike) : xbsIndex_r4/Delay  rst=off  infoeditControl=Selection of Reset will increase slice count due to use of real FFs and instead of SRLs  en=off  latency=1  reg_retiming=off  dbl_ovrd=off  block_type=delay
  Mult{,15..30} (17 alike) : xbsIndex_r4/Mult  precision=User Defined  arith_type="Signed  (2's comp)"  n_bits=W  bin_pt=B  quantization="Round  (unbiased: +/- Inf)"  overflow=Flag as error  en=off  latency=0  use_behavioral_HDL=off  opt=Speed  use_embedded=on  optimum_pipeline=off  pipeline=on  dbl_ovrd=off  use_rpm=on  placement_style=Triangular  block_type=mult
  Out1 : Outport
  wires:
  AddSub2/1 -> Out1/1
  Constant14/1 -> Mult16/2
  Mult/1 -> AddSub16/2
  Mult16/1 -> AddSub1/2
  AddSub16/1 -> Delay15/1
  Constant15/1 -> Mult/2
  AddSub1/1 -> Delay2/1
  Constant13/1 -> Mult17/2
  Mult17/1 -> AddSub18/2
  Constant12/1 -> Mult18/2
  AddSub17/1 -> Delay4/1
  AddSub18/1 -> Delay3/1
  Constant11/1 -> Mult19/2
  Mult19/1 -> AddSub20/2
  Constant10/1 -> Mult20/2
  Mult20/1 -> AddSub19/2
  AddSub19/1 -> Delay6/1
  AddSub20/1 -> Delay5/1
  Constant9/1 -> Mult21/2
  Mult21/1 -> AddSub22/2
  Constant8/1 -> Mult22/2
  AddSub21/1 -> Delay8/1
  AddSub22/1 -> Delay7/1
  Constant7/1 -> Mult23/2
  Mult23/1 -> AddSub24/2
  Constant6/1 -> Mult24/2
  AddSub23/1 -> Delay10/1
  Constant5/1 -> Mult25/2
  Mult25/1 -> AddSub26/2
  Constant4/1 -> Mult26/2
  Mult26/1 -> AddSub25/2
  AddSub25/1 -> Delay12/1
  AddSub26/1 -> Delay11/1
  Constant3/1 -> Mult27/2
  Mult27/1 -> AddSub28/2
  Constant2/1 -> Mult28/2
  AddSub27/1 -> Delay14/1
  AddSub28/1 -> Delay13/1
  Constant1/1 -> Mult29/2
  Mult29/1 -> AddSub30/2
  Constant/1 -> Mult30/2
  Mult30/1 -> Delay17/1
  AddSub30/1 -> Delay16/1
  AddSub24/1 -> Delay9/1
  Delay2/1 -> AddSub16/1
  Delay3/1 -> AddSub1/1
  Delay4/1 -> AddSub18/1
  Delay6/1 -> AddSub20/1
  Delay7/1 -> AddSub19/1
  Delay8/1 -> AddSub22/1
  Delay10/1 -> AddSub24/1
  Delay12/1 -> AddSub26/1
  Delay13/1 -> AddSub25/1
  Delay14/1 -> AddSub28/1
  Delay17/1 -> AddSub30/1
  Constant16/1 -> Mult15/2
  Mult15/1 -> AddSub2/2
  Delay15/1 -> AddSub2/1
  Delay5/1 -> AddSub17/1
  Mult18/1 -> AddSub17/2
  Delay9/1 -> AddSub21/1
  Mult22/1 -> AddSub21/2
  Delay11/1 -> AddSub23/1
  Mult24/1 -> AddSub23/2
  Delay16/1 -> AddSub27/1
  Mult28/1 -> AddSub27/2
  In1/1 -> Mult30/1, Mult29/1, Mult28/1, Mult27/1, Mult26/1, Mult25/1, Mult24/1, Mult22/1, Mult21/1, Mult19/1, Mult17/1, Mult15/1, Mult/1, Mult16/1, Mult18/1, Mult20/1, Mult23/1

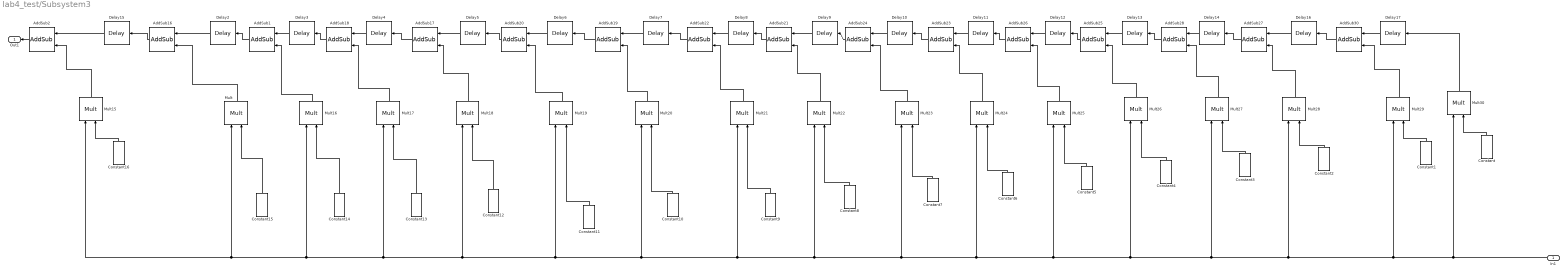
== system lab4_test/Subsystem3 ==
  In1 : Inport
  AddSub{1..2,16..28,30} (16 alike) : xbsIndex_r4/AddSub  mode=Addition  use_carryin=off  use_carryout=off  en=off  latency=0  precision=User Defined  arith_type="Signed  (2's comp)"  n_bits=W  bin_pt=B  quantization=Truncate  overflow=Wrap  use_behavioral_HDL=off  hw_selection=Fabric  pipelined=off  dbl_ovrd=off  block_type=addsub
  Constant : xbsIndex_r4/Constant  const=h(1,15)  gui_display_data_type=Fixed-point  arith_type=Signed (2's comp)  n_bits=W  bin_pt=B  preci_type=Single  exp_width=8  frac_width=24  explicit_period=off  period=1  equ=P=C  opselect=C  inp2=PCIN>>17  opr=+  inp1=P  carry=CIN  dbl_ovrd=off  block_type=constant
  Constant1 : xbsIndex_r4/Constant  const=h(2,15)  gui_display_data_type=Fixed-point  arith_type=Signed (2's comp)  n_bits=W  bin_pt=B  preci_type=Single  exp_width=8  frac_width=24  explicit_period=off  period=1  equ=P=C  opselect=C  inp2=PCIN>>17  opr=+  inp1=P  carry=CIN  dbl_ovrd=off  block_type=constant
  Constant10 : xbsIndex_r4/Constant  const=h(11,15)  gui_display_data_type=Fixed-point  arith_type=Signed (2's comp)  n_bits=W  bin_pt=B  preci_type=Single  exp_width=8  frac_width=24  explicit_period=off  period=1  equ=P=C  opselect=C  inp2=PCIN>>17  opr=+  inp1=P  carry=CIN  dbl_ovrd=off  block_type=constant
  Constant11 : xbsIndex_r4/Constant  const=h(12,15)  gui_display_data_type=Fixed-point  arith_type=Signed (2's comp)  n_bits=W  bin_pt=B  preci_type=Single  exp_width=8  frac_width=24  explicit_period=off  period=1  equ=P=C  opselect=C  inp2=PCIN>>17  opr=+  inp1=P  carry=CIN  dbl_ovrd=off  block_type=constant
  Constant12 : xbsIndex_r4/Constant  const=h(13,15)  gui_display_data_type=Fixed-point  arith_type=Signed (2's comp)  n_bits=W  bin_pt=B  preci_type=Single  exp_width=8  frac_width=24  explicit_period=off  period=1  equ=P=C  opselect=C  inp2=PCIN>>17  opr=+  inp1=P  carry=CIN  dbl_ovrd=off  block_type=constant
  Constant13 : xbsIndex_r4/Constant  const=h(14,15)  gui_display_data_type=Fixed-point  arith_type=Signed (2's comp)  n_bits=W  bin_pt=B  preci_type=Single  exp_width=8  frac_width=24  explicit_period=off  period=1  equ=P=C  opselect=C  inp2=PCIN>>17  opr=+  inp1=P  carry=CIN  dbl_ovrd=off  block_type=constant
  Constant14 : xbsIndex_r4/Constant  const=h(15,15)  gui_display_data_type=Fixed-point  arith_type=Signed (2's comp)  n_bits=W  bin_pt=B  preci_type=Single  exp_width=8  frac_width=24  explicit_period=off  period=1  equ=P=C  opselect=C  inp2=PCIN>>17  opr=+  inp1=P  carry=CIN  dbl_ovrd=off  block_type=constant
  Constant15 : xbsIndex_r4/Constant  const=h(16,15)  gui_display_data_type=Fixed-point  arith_type=Signed (2's comp)  n_bits=W  bin_pt=B  preci_type=Single  exp_width=8  frac_width=24  explicit_period=off  period=1  equ=P=C  opselect=C  inp2=PCIN>>17  opr=+  inp1=P  carry=CIN  dbl_ovrd=off  block_type=constant
  Constant16 : xbsIndex_r4/Constant  const=h(17,15)  gui_display_data_type=Fixed-point  arith_type=Signed (2's comp)  n_bits=W  bin_pt=B  preci_type=Single  exp_width=8  frac_width=24  explicit_period=off  period=1  equ=P=C  opselect=C  inp2=PCIN>>17  opr=+  inp1=P  carry=CIN  dbl_ovrd=off  block_type=constant
  Constant2 : xbsIndex_r4/Constant  const=h(3,15)  gui_display_data_type=Fixed-point  arith_type=Signed (2's comp)  n_bits=W  bin_pt=B  preci_type=Single  exp_width=8  frac_width=24  explicit_period=off  period=1  equ=P=C  opselect=C  inp2=PCIN>>17  opr=+  inp1=P  carry=CIN  dbl_ovrd=off  block_type=constant
  Constant3 : xbsIndex_r4/Constant  const=h(4,15)  gui_display_data_type=Fixed-point  arith_type=Signed (2's comp)  n_bits=W  bin_pt=B  preci_type=Single  exp_width=8  frac_width=24  explicit_period=off  period=1  equ=P=C  opselect=C  inp2=PCIN>>17  opr=+  inp1=P  carry=CIN  dbl_ovrd=off  block_type=constant
  Constant4 : xbsIndex_r4/Constant  const=h(5,15)  gui_display_data_type=Fixed-point  arith_type=Signed (2's comp)  n_bits=W  bin_pt=B  preci_type=Single  exp_width=8  frac_width=24  explicit_period=off  period=1  equ=P=C  opselect=C  inp2=PCIN>>17  opr=+  inp1=P  carry=CIN  dbl_ovrd=off  block_type=constant
  Constant5 : xbsIndex_r4/Constant  const=h(6,15)  gui_display_data_type=Fixed-point  arith_type=Signed (2's comp)  n_bits=W  bin_pt=B  preci_type=Single  exp_width=8  frac_width=24  explicit_period=off  period=1  equ=P=C  opselect=C  inp2=PCIN>>17  opr=+  inp1=P  carry=CIN  dbl_ovrd=off  block_type=constant
  Constant6 : xbsIndex_r4/Constant  const=h(7,15)  gui_display_data_type=Fixed-point  arith_type=Signed (2's comp)  n_bits=W  bin_pt=B  preci_type=Single  exp_width=8  frac_width=24  explicit_period=off  period=1  equ=P=C  opselect=C  inp2=PCIN>>17  opr=+  inp1=P  carry=CIN  dbl_ovrd=off  block_type=constant
  Constant7 : xbsIndex_r4/Constant  const=h(8,15)  gui_display_data_type=Fixed-point  arith_type=Signed (2's comp)  n_bits=W  bin_pt=B  preci_type=Single  exp_width=8  frac_width=24  explicit_period=off  period=1  equ=P=C  opselect=C  inp2=PCIN>>17  opr=+  inp1=P  carry=CIN  dbl_ovrd=off  block_type=constant
  Constant8 : xbsIndex_r4/Constant  const=h(9,15)  gui_display_data_type=Fixed-point  arith_type=Signed (2's comp)  n_bits=W  bin_pt=B  preci_type=Single  exp_width=8  frac_width=24  explicit_period=off  period=1  equ=P=C  opselect=C  inp2=PCIN>>17  opr=+  inp1=P  carry=CIN  dbl_ovrd=off  block_type=constant
  Constant9 : xbsIndex_r4/Constant  const=h(10,15)  gui_display_data_type=Fixed-point  arith_type=Signed (2's comp)  n_bits=W  bin_pt=B  preci_type=Single  exp_width=8  frac_width=24  explicit_period=off  period=1  equ=P=C  opselect=C  inp2=PCIN>>17  opr=+  inp1=P  carry=CIN  dbl_ovrd=off  block_type=constant
  Delay{2..17} (16 alike) : xbsIndex_r4/Delay  rst=off  infoeditControl=Selection of Reset will increase slice count due to use of real FFs and instead of SRLs  en=off  latency=1  reg_retiming=off  dbl_ovrd=off  block_type=delay
  Mult{,15..30} (17 alike) : xbsIndex_r4/Mult  precision=User Defined  arith_type="Signed  (2's comp)"  n_bits=W  bin_pt=B  quantization="Round  (unbiased: +/- Inf)"  overflow=Flag as error  en=off  latency=0  use_behavioral_HDL=off  opt=Speed  use_embedded=on  optimum_pipeline=off  pipeline=on  dbl_ovrd=off  use_rpm=on  placement_style=Triangular  block_type=mult
  Out1 : Outport
  wires:
  AddSub2/1 -> Out1/1
  Constant14/1 -> Mult16/2
  Mult/1 -> AddSub16/2
  Mult16/1 -> AddSub1/2
  AddSub16/1 -> Delay15/1
  Constant15/1 -> Mult/2
  AddSub1/1 -> Delay2/1
  Constant13/1 -> Mult17/2
  Mult17/1 -> AddSub18/2
  Constant12/1 -> Mult18/2
  AddSub17/1 -> Delay4/1
  AddSub18/1 -> Delay3/1
  Constant11/1 -> Mult19/2
  Mult19/1 -> AddSub20/2
  Constant10/1 -> Mult20/2
  Mult20/1 -> AddSub19/2
  AddSub19/1 -> Delay6/1
  AddSub20/1 -> Delay5/1
  Constant9/1 -> Mult21/2
  Mult21/1 -> AddSub22/2
  Constant8/1 -> Mult22/2
  AddSub21/1 -> Delay8/1
  AddSub22/1 -> Delay7/1
  Constant7/1 -> Mult23/2
  Mult23/1 -> AddSub24/2
  Constant6/1 -> Mult24/2
  AddSub23/1 -> Delay10/1
  Constant5/1 -> Mult25/2
  Mult25/1 -> AddSub26/2
  Constant4/1 -> Mult26/2
  Mult26/1 -> AddSub25/2
  AddSub25/1 -> Delay12/1
  AddSub26/1 -> Delay11/1
  Constant3/1 -> Mult27/2
  Mult27/1 -> AddSub28/2
  Constant2/1 -> Mult28/2
  AddSub27/1 -> Delay14/1
  AddSub28/1 -> Delay13/1
  Constant1/1 -> Mult29/2
  Mult29/1 -> AddSub30/2
  Constant/1 -> Mult30/2
  Mult30/1 -> Delay17/1
  AddSub30/1 -> Delay16/1
  AddSub24/1 -> Delay9/1
  Delay2/1 -> AddSub16/1
  Delay3/1 -> AddSub1/1
  Delay4/1 -> AddSub18/1
  Delay6/1 -> AddSub20/1
  Delay7/1 -> AddSub19/1
  Delay8/1 -> AddSub22/1
  Delay10/1 -> AddSub24/1
  Delay12/1 -> AddSub26/1
  Delay13/1 -> AddSub25/1
  Delay14/1 -> AddSub28/1
  Delay17/1 -> AddSub30/1
  Constant16/1 -> Mult15/2
  Mult15/1 -> AddSub2/2
  Delay15/1 -> AddSub2/1
  Delay5/1 -> AddSub17/1
  Mult18/1 -> AddSub17/2
  Delay9/1 -> AddSub21/1
  Mult22/1 -> AddSub21/2
  Delay11/1 -> AddSub23/1
  Mult24/1 -> AddSub23/2
  Delay16/1 -> AddSub27/1
  Mult28/1 -> AddSub27/2
  In1/1 -> Mult30/1, Mult29/1, Mult28/1, Mult27/1, Mult26/1, Mult25/1, Mult24/1, Mult22/1, Mult21/1, Mult19/1, Mult17/1, Mult15/1, Mult/1, Mult16/1, Mult18/1, Mult20/1, Mult23/1
